simulink model "fungerande200ka"  (R2017a)
settings: Solver=VariableStepAuto  StartTime=0.0  StopTime=0.0015  RelTol=1e-3
libraries: fl_lib x30, nesl_utility x8, elec_lib x4
settings Model: Creator=nippe  LastModifiedBy=Frans
settings OptimizationCC: LifeSpan=inf
settings DebuggingCC: SFExecutionAtInitializationDiag=none

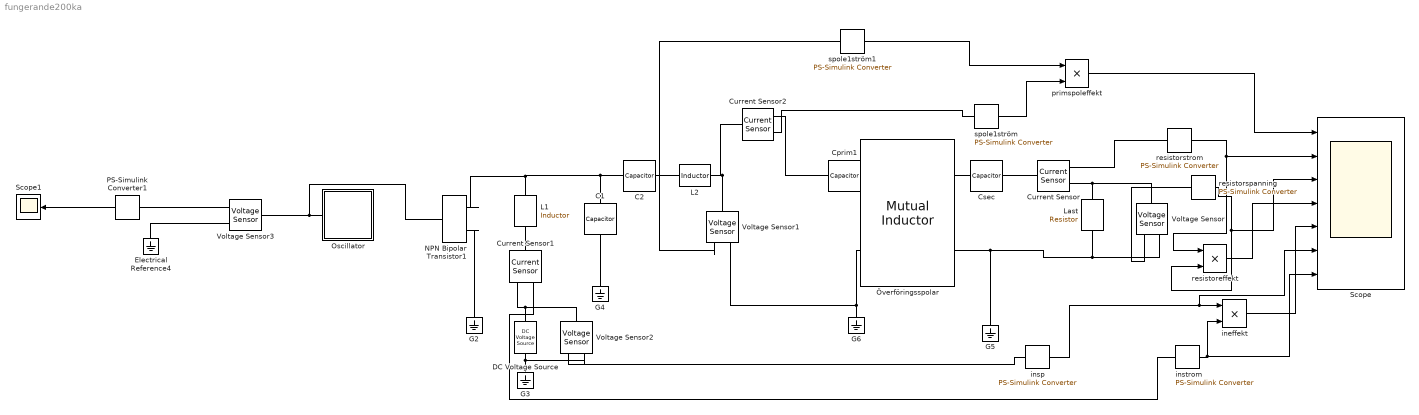
== system fungerande200ka ==
  C1 : fl_lib/Electrical/Electrical Elements/Capacitor  c=24.29841304777091 nF  r=1e-6 Ohm  g=0 1/Ohm  i_specify=off  i_priority=None  i=0 A  i_nominal_specify=off  i_nominal_unit=A  i_nominal_value=1  v_specify=off  v_priority=None  v=0 V  v_nominal_specify=off  v_nominal_unit=V  v_nominal_value=1  vc_specify=off  vc_priority=High  vc=0 V  vc_nominal_specify=off  vc_nominal_unit=V  vc_nominal_value=1
  C2 : fl_lib/Electrical/Electrical Elements/Capacitor  c=8.809942539470194 nF  r=1e-6 Ohm  g=0 1/Ohm  i_specify=off  i_priority=None  i=0 A  i_nominal_specify=off  i_nominal_unit=A  i_nominal_value=1  v_specify=off  v_priority=None  v=0 V  v_nominal_specify=off  v_nominal_unit=V  v_nominal_value=1  vc_specify=off  vc_priority=High  vc=0 V  vc_nominal_specify=off  vc_nominal_unit=V  vc_nominal_value=1
  Cprim1 : fl_lib/Electrical/Electrical Elements/Capacitor  c=6.1303 nF  r=0.074 Ohm  g=0 1/Ohm  i_specify=off  i_priority=None  i=0 A  i_nominal_specify=off  i_nominal_unit=A  i_nominal_value=1  v_specify=off  v_priority=None  v=0 V  v_nominal_specify=off  v_nominal_unit=V  v_nominal_value=1  vc_specify=off  vc_priority=High  vc=0 V  vc_nominal_specify=off  vc_nominal_unit=V  vc_nominal_value=1
  Csec : fl_lib/Electrical/Electrical Elements/Capacitor  c=6.1303 nF  r=0.074 Ohm  g=0 1/Ohm  i_specify=off  i_priority=None  i=0 A  i_nominal_specify=off  i_nominal_unit=A  i_nominal_value=1  v_specify=off  v_priority=None  v=0 V  v_nominal_specify=off  v_nominal_unit=V  v_nominal_value=1  vc_specify=off  vc_priority=High  vc=0 V  vc_nominal_specify=off  vc_nominal_unit=V  vc_nominal_value=1
  Current Sensor : fl_lib/Electrical/Electrical Sensors/Current Sensor
  Current Sensor1 : fl_lib/Electrical/Electrical Sensors/Current Sensor
  Current Sensor2 : fl_lib/Electrical/Electrical Sensors/Current Sensor
  DC Voltage Source : fl_lib/Electrical/Electrical Sources/DC Voltage Source  v0=25 V
  Electrical Reference4 : fl_lib/Electrical/Electrical Elements/Electrical Reference
  G{2..6} (5 alike) : fl_lib/Electrical/Electrical Elements/Electrical Reference
  L1 : fl_lib/Electrical/Electrical Elements/Inductor  l=1 mH  r=1 Ohm  g=1e-9 1/Ohm  i_specify=off  i_priority=None  i=0 A  i_nominal_specify=off  i_nominal_unit=A  i_nominal_value=1  v_specify=off  v_priority=None  v=0 V  v_nominal_specify=off  v_nominal_unit=V  v_nominal_value=1  i_L_specify=off  i_L_priority=High  i_L=0 A  i_L_nominal_specify=off  i_L_nominal_unit=A  i_L_nominal_value=1
  L2 : fl_lib/Electrical/Electrical Elements/Inductor  l=76.92656502356618 uH  r=0.015 Ohm  g=1e-9 1/Ohm  i_specify=off  i_priority=None  i=0 A  i_nominal_specify=off  i_nominal_unit=A  i_nominal_value=1  v_specify=off  v_priority=None  v=0 V  v_nominal_specify=off  v_nominal_unit=V  v_nominal_value=1  i_L_specify=off  i_L_priority=High  i_L=0 A  i_L_nominal_specify=off  i_L_nominal_unit=A  i_L_nominal_value=1
  Last : fl_lib/Electrical/Electrical Elements/Resistor  R=29.45 Ohm  i_specify=off  i_priority=None  i=0 A  i_nominal_specify=off  i_nominal_unit=A  i_nominal_value=1  v_specify=off  v_priority=None  v=0 V  v_nominal_specify=off  v_nominal_unit=V  v_nominal_value=1
  NPN Bipolar Transistor1 : elec_lib/Semiconductor Devices/NPN Bipolar Transistor  parameterization=1  prmDatasheet=1  prmEquCoeff=1  BF=100  IS=1e-14 A  ec=1  VAF=200 V  hfe=100  hoe=5e-5 1/Ohm  Ic_h=1 mA  Vce_h=5 V  V1=1 V  I1=0.5 mA  BR=1  Tmeas=25 degC  RC=0.01 Ohm  RE=1e-4 Ohm  RB=1 Ohm  C_BC=5 pF  C_BE=5 pF  TF=0 us  TR=0 us  hfe_T2=125  XTB=0  V1_T2=0.45 V  I1_T2=0.5 mA  Tmeas2=125 degC  EG=1.11 eV  XTI=3  TdeviceDatasheet=25 degC  TdeviceEquCoeff=25 degC  Rth=[ 0 10 ] K/W  thermal_mass_parameterization=1  thermal_mass=[ 0 1 ] J/K  thermal_time_constant=[ 0 10 ] s  thermal_mass_initial_temperatures=[ 25 25 ] degC
      settings: SourceProductName=Simscape Electronics  SourceProductBaseCode=SN
  Oscillator : Subsystem
  PS-Simulink Converter1 : nesl_utility/PS-Simulink Converter  PhysicalDomain=network_engine_domain  SubClassName=ps_output  LeftPortType=input  RightPortType=output  PseudoPeriodic=off  Frequencies=[]  Unit=1  AffineConversion=off
  Scope : Scope  NumInputPorts=7
  Scope1 : Scope
  Voltage Sensor{,1..3} (4 alike) : fl_lib/Electrical/Electrical Sensors/Voltage Sensor
  ineffekt : Product
  insp : nesl_utility/PS-Simulink Converter  PhysicalDomain=network_engine_domain  SubClassName=ps_output  LeftPortType=input  RightPortType=output  PseudoPeriodic=off  Frequencies=[]  Unit=1  AffineConversion=off
  instrom : nesl_utility/PS-Simulink Converter  PhysicalDomain=network_engine_domain  SubClassName=ps_output  LeftPortType=input  RightPortType=output  PseudoPeriodic=off  Frequencies=[]  Unit=1  AffineConversion=off
  primspoleffekt : Product
  "resistoreffekt " : Product
  resistorspanning : nesl_utility/PS-Simulink Converter  PhysicalDomain=network_engine_domain  SubClassName=ps_output  LeftPortType=input  RightPortType=output  PseudoPeriodic=off  Frequencies=[]  Unit=1  AffineConversion=off
  resistorstrom : nesl_utility/PS-Simulink Converter  PhysicalDomain=network_engine_domain  SubClassName=ps_output  LeftPortType=input  RightPortType=output  PseudoPeriodic=off  Frequencies=[]  Unit=1  AffineConversion=off
  spole1ström : nesl_utility/PS-Simulink Converter  PhysicalDomain=network_engine_domain  SubClassName=ps_output  LeftPortType=input  RightPortType=output  PseudoPeriodic=off  Frequencies=[]  Unit=1  AffineConversion=off
  spole1ström1 : nesl_utility/PS-Simulink Converter  PhysicalDomain=network_engine_domain  SubClassName=ps_output  LeftPortType=input  RightPortType=output  PseudoPeriodic=off  Frequencies=[]  Unit=1  AffineConversion=off
  Överföringsspolar : fl_lib/Electrical/Electrical Elements/Mutual Inductor  L1=1.0330e-04 H  L2=1.0330e-04 H  k=0.10635043562  i1_specify=off  i1_priority=High  i1=0 A  i1_nominal_specify=off  i1_nominal_unit=A  i1_nominal_value=1  i2_specify=off  i2_priority=High  i2=0 A  i2_nominal_specify=off  i2_nominal_unit=A  i2_nominal_value=1  v1_specify=off  v1_priority=None  v1=0 V  v1_nominal_specify=off  v1_nominal_unit=V  v1_nominal_value=1  v2_specify=off  v2_priority=None  v2=0 V  v2_nominal_specify=off  v2_nominal_unit=V  v2_nominal_value=1
      settings: SourceProductName=Simscape  SourceProductBaseCode=SS
  wires:
  resistorspanning/1 -> "resistoreffekt "/2, Scope/3
  resistorstrom/1 -> "resistoreffekt "/1, Scope/2
  "resistoreffekt "/1 -> Scope/4
  ineffekt/1 -> Scope/5
  instrom/1 -> Scope/7, ineffekt/2
  insp/1 -> ineffekt/1, Scope/6
  spole1ström1/1 -> primspoleffekt/1
  PS-Simulink Converter1/1 -> Scope1/1
  spole1ström/1 -> primspoleffekt/2
  primspoleffekt/1 -> Scope/1
  connections:
  L2/LConn1 -- C2/RConn1
  Voltage Sensor/LConn1 -- Current Sensor/RConn2 -- Last/LConn1
  C2/LConn1 -- C1/LConn1 -- NPN Bipolar Transistor1/RConn1 -- L1/RConn1
  G4/LConn1 -- C1/RConn1
  Voltage Sensor/RConn1 -- resistorspanning/LConn1
  G3/LConn1 -- Voltage Sensor2/RConn2 -- DC Voltage Source/RConn1
  NPN Bipolar Transistor1/RConn2 -- G2/LConn1
  Csec/LConn1 -- Överföringsspolar/RConn1
  Csec/RConn1 -- Current Sensor/LConn1
  Current Sensor/RConn1 -- resistorstrom/LConn1
  G6/LConn1 -- Voltage Sensor1/RConn2 -- Överföringsspolar/LConn2
  Voltage Sensor/RConn2 -- G5/LConn1 -- Överföringsspolar/RConn2 -- Last/RConn1
  L1/LConn1 -- Current Sensor1/LConn1
  Current Sensor1/RConn2 -- Voltage Sensor2/LConn1 -- DC Voltage Source/LConn1
  Current Sensor1/RConn1 -- instrom/LConn1
  Voltage Sensor2/RConn1 -- insp/LConn1
  spole1ström/LConn1 -- Current Sensor2/RConn1
  Voltage Sensor1/RConn1 -- spole1ström1/LConn1
  Cprim1/LConn1 -- Överföringsspolar/LConn1
  Voltage Sensor3/RConn1 -- PS-Simulink Converter1/LConn1
  Voltage Sensor3/RConn2 -- Electrical Reference4/LConn1
  NPN Bipolar Transistor1/LConn1 -- Voltage Sensor3/LConn1 -- Oscillator/LConn1
  Current Sensor2/RConn2 -- Cprim1/RConn1
  Current Sensor2/LConn1 -- L2/RConn1 -- Voltage Sensor1/LConn1

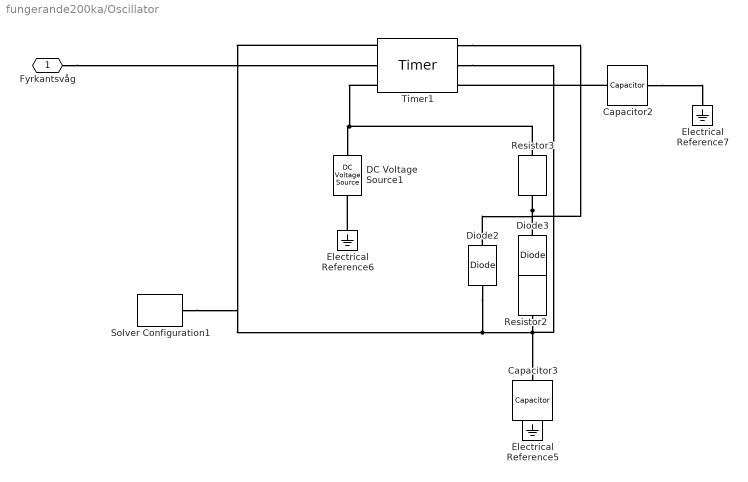
== system fungerande200ka/Oscillator ==
  Capacitor2 : fl_lib/Electrical/Electrical Elements/Capacitor  c=1e-8 F  r=1e-6 Ohm  g=0 1/Ohm  i_specify=off  i_priority=None  i=0 A  i_nominal_specify=off  i_nominal_unit=A  i_nominal_value=1  v_specify=off  v_priority=None  v=0 V  v_nominal_specify=off  v_nominal_unit=V  v_nominal_value=1  vc_specify=off  vc_priority=High  vc=0 V  vc_nominal_specify=off  vc_nominal_unit=V  vc_nominal_value=1
  Capacitor3 : fl_lib/Electrical/Electrical Elements/Capacitor  c=1e-8 F  r=1e-6 Ohm  g=0 1/Ohm  i_specify=off  i_priority=None  i=0 A  i_nominal_specify=off  i_nominal_unit=A  i_nominal_value=1  v_specify=off  v_priority=None  v=0 V  v_nominal_specify=off  v_nominal_unit=V  v_nominal_value=1  vc_specify=off  vc_priority=High  vc=0 V  vc_nominal_specify=off  vc_nominal_unit=V  vc_nominal_value=1
  DC Voltage Source1 : fl_lib/Electrical/Electrical Sources/DC Voltage Source  v0=3 V
  Diode2 : elec_lib/Semiconductor Devices/Diode  ModelType=1  Vf=0.1 V  Ron=0.1 Ohm  Goff=1e-8 S  Rz=0.3 Ohm  Vz=50 V  C_PWL=0 pF  prmExp=1  I12=[0.0137, 0.545] A  V12=[0.6, 0.7] V  I1=0.0137 A  V1=0.6 V  IS=1e-12 A  ec=1  RS=0.01 Ohm  Tmeas=25 degC  BV=inf V  C_param=1  CJ0=5 pF  VJ=1 V  Mgrad=0.5  Vvec=[0.1, 10.0, 100.0] V  Cvec=[3.5, 1.0, 0.4] pF  FC=0.5  Q_param=1  Irrm=-7.15 A  iF=4 A  didt=-750 A/us  trr=115 ns  TT=50 ns  tau=100 ns  T_param=1  IS_T2=1.25e-7 A  I1_T2=0.245 A  V1_T2=0.5 V  Tmeas2=125 degC  EG_param=1  EG=1.11 eV  XTI_param=1  XTI=3  dBVdT=0 V/K  Tdevice=25 degC  i_capacitor_specify=off  i_capacitor_priority=High  i_capacitor=0 A  i_capacitor_nominal_specify=off  i_capacitor_nominal_unit=A  i_capacitor_nominal_value=1  v_capacitor_specify=off  v_capacitor_priority=None  v_capacitor=0 V  v_capacitor_nominal_specify=off  v_capacitor_nominal_unit=V  v_capacitor_nominal_value=1  Rth=[0.0, 10.0] K/W  thermal_mass_parameterization=1  thermal_mass=[0.0, 1.0] J/K  thermal_time_constant=[0.0, 10.0] s  thermal_mass_initial_temperatures=[25.0, 25.0] degC
      settings: SourceProductName=Simscape Electronics  SourceProductBaseCode=SN
  Diode3 : elec_lib/Semiconductor Devices/Diode  ModelType=1  Vf=0.1 V  Ron=0.1 Ohm  Goff=1e-8 S  Rz=0.3 Ohm  Vz=50 V  C_PWL=0 pF  prmExp=1  I12=[0.0137, 0.545] A  V12=[0.6, 0.7] V  I1=0.0137 A  V1=0.6 V  IS=1e-12 A  ec=1  RS=0.01 Ohm  Tmeas=25 degC  BV=inf V  C_param=1  CJ0=5 pF  VJ=1 V  Mgrad=0.5  Vvec=[0.1, 10.0, 100.0] V  Cvec=[3.5, 1.0, 0.4] pF  FC=0.5  Q_param=1  Irrm=-7.15 A  iF=4 A  didt=-750 A/us  trr=115 ns  TT=50 ns  tau=100 ns  T_param=1  IS_T2=1.25e-7 A  I1_T2=0.245 A  V1_T2=0.5 V  Tmeas2=125 degC  EG_param=1  EG=1.11 eV  XTI_param=1  XTI=3  dBVdT=0 V/K  Tdevice=25 degC  i_capacitor_specify=off  i_capacitor_priority=High  i_capacitor=0 A  i_capacitor_nominal_specify=off  i_capacitor_nominal_unit=A  i_capacitor_nominal_value=1  v_capacitor_specify=off  v_capacitor_priority=None  v_capacitor=0 V  v_capacitor_nominal_specify=off  v_capacitor_nominal_unit=V  v_capacitor_nominal_value=1  Rth=[0.0, 10.0] K/W  thermal_mass_parameterization=1  thermal_mass=[0.0, 1.0] J/K  thermal_time_constant=[0.0, 10.0] s  thermal_mass_initial_temperatures=[25.0, 25.0] degC
      settings: SourceProductName=Simscape Electronics  SourceProductBaseCode=SN
  Electrical Reference5 : fl_lib/Electrical/Electrical Elements/Electrical Reference
  Electrical Reference6 : fl_lib/Electrical/Electrical Elements/Electrical Reference
  Electrical Reference7 : fl_lib/Electrical/Electrical Elements/Electrical Reference
  Resistor2 : fl_lib/Electrical/Electrical Elements/Resistor  R=282 Ohm  i_specify=off  i_priority=None  i=0 A  i_nominal_specify=off  i_nominal_unit=A  i_nominal_value=1  v_specify=off  v_priority=None  v=0 V  v_nominal_specify=off  v_nominal_unit=V  v_nominal_value=1
  Resistor3 : fl_lib/Electrical/Electrical Elements/Resistor  R=322 Ohm  i_specify=off  i_priority=None  i=0 A  i_nominal_specify=off  i_nominal_unit=A  i_nominal_value=1  v_specify=off  v_priority=None  v=0 V  v_nominal_specify=off  v_nominal_unit=V  v_nominal_value=1
  Solver Configuration1 : nesl_utility/Solver Configuration  PhysicalDomain=network_engine_domain  SubClassName=solver  LeftPortType=input  RightPortType=generic  Accelerate=off  Tones=[]  Harmonics=[]  SimulateNoise=off  Profile=off  UseLocalSampling=off  EnableSwitchedLinearOptims=on  FrequencyDomain=off  UseCCode=off  RelTol=0.001  AbsTol=1e-06  MinStep=1e-09  ToWorkspace=off  RevertToSquareIcSolve=off  NumHomotopyIterations=100  PhasorMode=off  PhasorModeNumHarmonics=1  OverrideAbsTol=off  DoDC=off  ResidualTolerance=1e-09  UseLocalSolver=off  LocalSolverChoice=NE_BACKWARD_EULER_ADVANCER  LocalSolverSampleTime=0.001  DoFixedCost=off  MaxNonlinIter=3  MaxModeIter=2  LinearAlgebra=Sparse  DelaysMemoryBudget=1024  AutomaticFiltering=on  FilteringTimeConstant=0.001
  Timer1 : elec_lib/Integrated Circuits/Timer  V_CC=3 V  V_OL=0 V  V_OH=3 V  R_OUT=8 Ohm  Delay=1e-7 s  R_DIV=5 kOhm  R_closed=12 Ohm  R_open=5e+8 Ohm
      settings: SourceProductName=Simscape Electronics  SourceProductBaseCode=SN
  Fyrkantsvåg : PMIOPort  Port=1  Side=Left
  connections:
  Capacitor2/LConn1 -- Timer1/RConn3
  Fyrkantsvåg/RConn1 -- Timer1/LConn2
  Electrical Reference5/LConn1 -- Capacitor3/RConn1
  Resistor3/RConn1 -- Diode2/LConn1 -- Diode3/RConn1 -- Timer1/RConn1
  Resistor3/LConn1 -- Timer1/LConn3 -- DC Voltage Source1/LConn1
  Timer1/RConn2 -- Resistor2/RConn1 -- Solver Configuration1/RConn1 -- Timer1/LConn1 -- Diode2/RConn1 -- Capacitor3/LConn1
  Capacitor2/RConn1 -- Electrical Reference7/LConn1
  Diode3/LConn1 -- Resistor2/LConn1
  Electrical Reference6/LConn1 -- DC Voltage Source1/RConn1
